simulink model "MRAC_Gradiet_LS_Algorithm_Ex8"  (R2023a)
settings: Solver=VariableStepAuto  StartTime=0.0  StopTime=20.0  RelTol=1e-13  AbsTol=1e-10
undefined symbols (not defined in the file): a, b, gamma1, gamma2, r0, r1
libraries: dspinverses x1, dspfactors x1
settings Model: Creator=geokr  LastModifiedBy=geokr

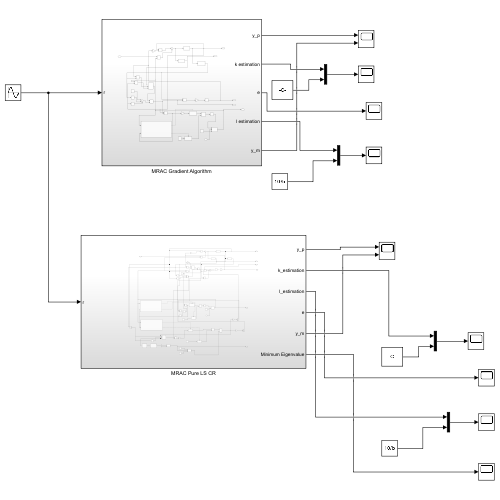
[thumbnail: Simulink's stored preview of the top-level diagram]
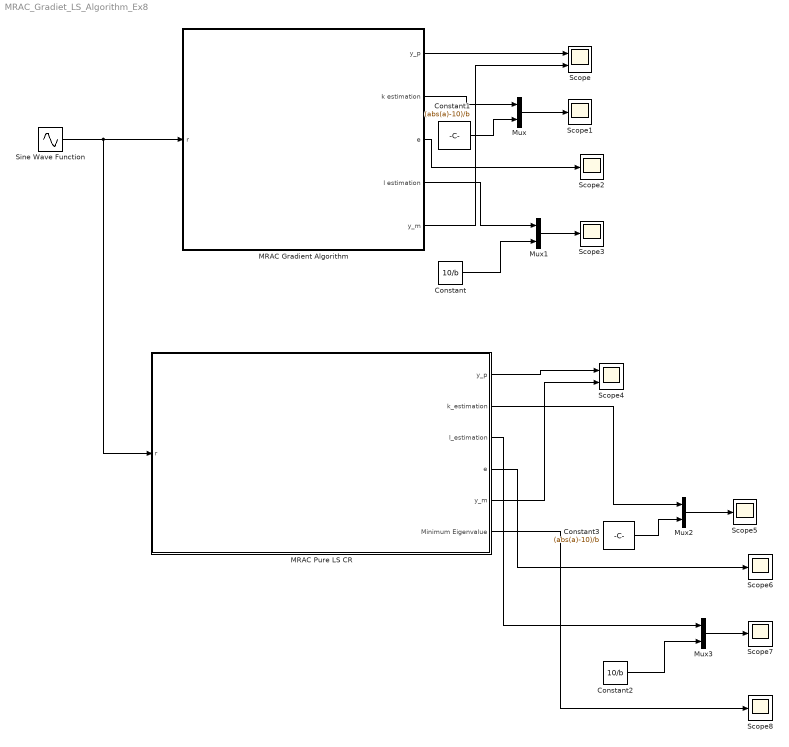
== system MRAC_Gradiet_LS_Algorithm_Ex8 ==
  Constant : Constant  Value=10/b
  Constant1 : Constant  Value=(abs(a)-10)/b
  Constant2 : Constant  Value=10/b
  Constant3 : Constant  Value=(abs(a)-10)/b
  MRAC Gradient Algorithm : Subsystem
  MRAC Pure LS CR : Subsystem
  Mux{,1..3} (4 alike) : Mux  Inputs=2
  Scope : Scope  NumInputPorts=2
  Scope{1..3,5..8} (7 alike) : Scope
  Scope4 : Scope  NumInputPorts=2
  Sine Wave Function : Sin  Frequency=2  SampleTime=0
  wires:
  MRAC Gradient Algorithm/1(y_p) -> Scope/1
  MRAC Gradient Algorithm/3(e) -> Scope2/1
  Mux/1 -> Scope1/1
  Mux1/1 -> Scope3/1
  MRAC Gradient Algorithm/2(k estimation) -> Mux/1
  MRAC Gradient Algorithm/4(l estimation) -> Mux1/1
  Constant/1 -> Mux1/2
  Constant1/1 -> Mux/2
  Sine Wave Function/1 -> MRAC Pure LS CR/1(r), MRAC Gradient Algorithm/1(r)
  MRAC Gradient Algorithm/5(y_m) -> Scope/2
  MRAC Pure LS CR/1(y_p) -> Scope4/1
  Constant3/1 -> Mux2/2
  Mux2/1 -> Scope5/1
  MRAC Pure LS CR/2(k_estimation) -> Mux2/1
  Mux3/1 -> Scope7/1
  Constant2/1 -> Mux3/2
  MRAC Pure LS CR/3(l_estimation) -> Mux3/1
  MRAC Pure LS CR/5(y_m) -> Scope4/2
  MRAC Pure LS CR/4(e) -> Scope6/1
  MRAC Pure LS CR/6(Minimum Eigenvalue) -> Scope8/1

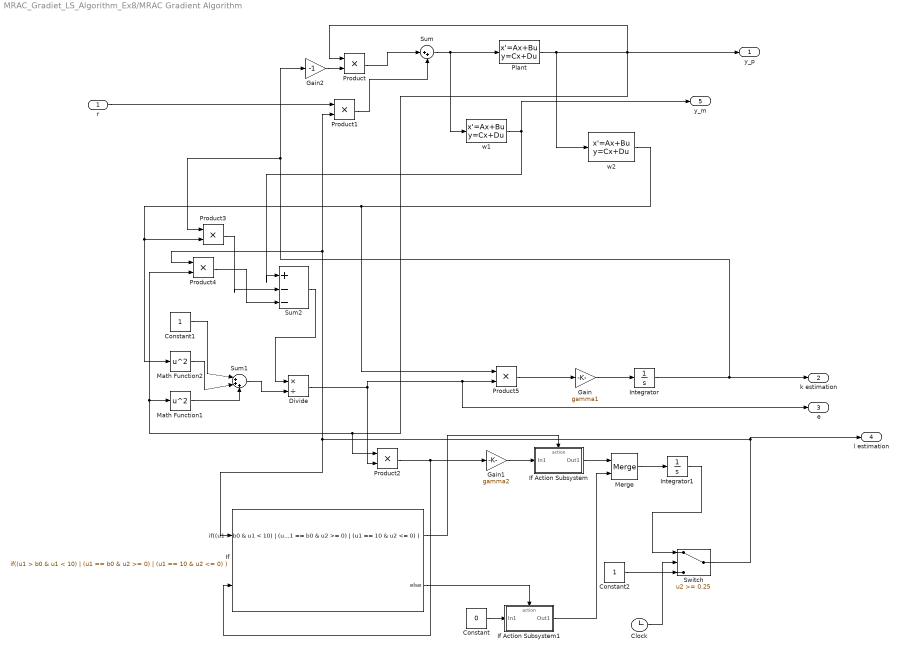
== system MRAC_Gradiet_LS_Algorithm_Ex8/MRAC Gradient Algorithm ==
  r : Inport
  Clock : Clock
  Constant : Constant  Value=0
  Constant1 : Constant
  Constant2 : Constant
  Divide : Product  Inputs=*/
  Gain : Gain  Gain=gamma1
  Gain1 : Gain  Gain=gamma2
  Gain2 : Gain  Gain=-1
  If : If  NumInputs=2  IfExpression=(u1 > b0 & u1 < 10) | (u1 == b0 & u2 >= 0) | (u1 == 10 & u2 <= 0)
  If Action Subsystem : Subsystem  TreatAsAtomicUnit=on
  If Action Subsystem1 : Subsystem  TreatAsAtomicUnit=on
  Integrator : Integrator
  Integrator1 : Integrator
  Math Function1 : Math  Operator=square
  Math Function2 : Math  Operator=square
  Merge : Merge
  Plant : StateSpace  A=a  B=b  D=0  InitialCondition=0
  Product{,1..5} (6 alike) : Product
  Sum : Sum  Inputs=|++
  Sum1 : Sum  Inputs=|+++
  Sum2 : Sum  Inputs=|+--
  Switch : Switch  Threshold=0.25  SaturateOnIntegerOverflow=off  InputSameDT=off
  w1 : StateSpace  A=-10  B=10  D=0  InitialCondition=0
  w2 : StateSpace  A=-10  B=10  D=0  InitialCondition=0
  y_p : Outport
  k estimation : Outport  Port=2
  e : Outport  Port=3
  l estimation : Outport  Port=4
  y_m : Outport  Port=5
  wires:
  If Action Subsystem/1(Out1) -> Merge/1
  Product2/1 -> If/2, Gain1/1
  Math Function2/1 -> Sum1/2
  Product/1 -> Sum/1
  w2/1 -> Math Function2/1, Product3/2, Product5/1
  Plant/1 -> w2/1, Product2/1, Product4/2, Math Function1/1, y_p/1, Product/1
  r/1 -> Product1/1
  Sum/1 -> w1/1, Plant/1
  Gain/1 -> Integrator/1
  Constant/1 -> If Action Subsystem1/1(In1)
  Math Function1/1 -> Sum1/3
  Product1/1 -> Sum/2
  w1/1 -> y_m/1, Sum2/1
  Gain1/1 -> If Action Subsystem/1(In1)
  If/2 -> If Action Subsystem1/Action
  Product3/1 -> Sum2/2
  If/1 -> If Action Subsystem/Action
  If Action Subsystem1/1(Out1) -> Merge/2
  Constant1/1 -> Sum1/1
  Product4/1 -> Sum2/3
  Sum1/1 -> Divide/2
  Product5/1 -> Gain/1
  Clock/1 -> Switch/2
  Merge/1 -> Integrator1/1
  Switch/1 -> If/1, Product4/1, Product1/2, l estimation/1
  Constant2/1 -> Switch/3
  Integrator1/1 -> Switch/1
  Integrator/1 -> k estimation/1, Gain2/1, Product3/1
  Sum2/1 -> Divide/1
  Divide/1 -> Product2/2, Product5/2, e/1
  Gain2/1 -> Product/2

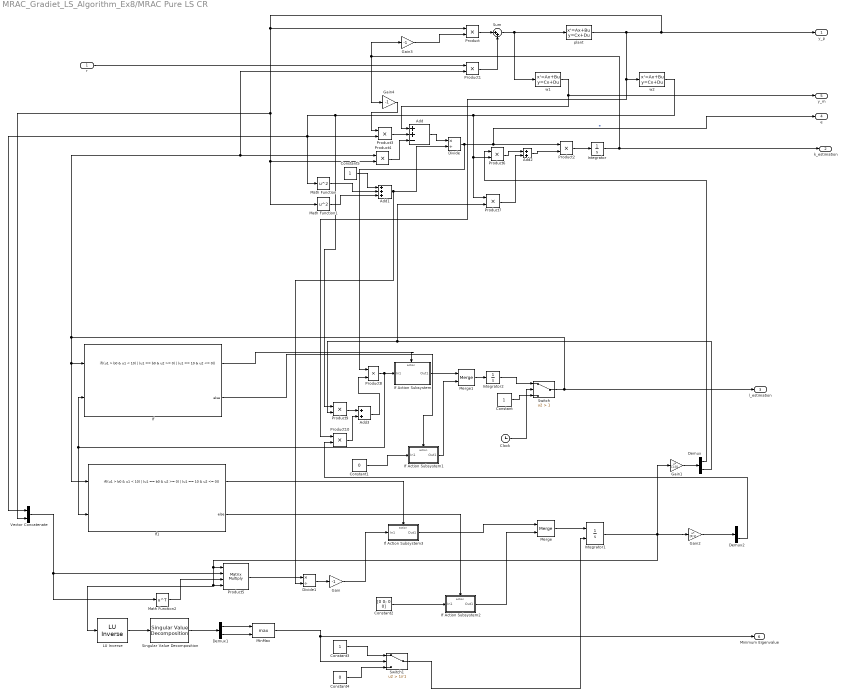
== system MRAC_Gradiet_LS_Algorithm_Ex8/MRAC Pure LS CR ==
  r : Inport
  " LU Inverse" : dspinverses/ LU Inverse
  Add : Sum  Inputs=++-
  Add1 : Sum  Inputs=+++
  Add2 : Sum
  Add3 : Sum
  Clock : Clock
  Constant : Constant
  Constant1 : Constant  Value=0
  Constant2 : Constant  Value=[0 0; 0 0]
  Constant3 : Constant
  Constant4 : Constant  Value=0
  Constant5 : Constant
  Demux : Demux  Outputs=2
  Demux1 : Demux  Outputs=2
  Demux2 : Demux  Outputs=2
  Divide : Product  Inputs=*/
  Divide1 : Product  Inputs=*/
  Gain : Gain  Gain=-1
  Gain1 : Gain  Gain=[1;0]  Multiplication=Matrix(u*K)
  Gain2 : Gain  Gain=[0;1]  Multiplication=Matrix(u*K)
  Gain3 : Gain  Gain=-1
  Gain4 : Gain  Gain=-1
  If : If  NumInputs=2  IfExpression=(u1 > b0 & u1 < 10) | (u1 == b0 & u2 >= 0) | (u1 == 10 & u2 <= 0)
  If Action Subsystem : Subsystem  TreatAsAtomicUnit=on
  If Action Subsystem1 : Subsystem  TreatAsAtomicUnit=on
  If Action Subsystem2 : Subsystem  TreatAsAtomicUnit=on
  If Action Subsystem3 : Subsystem  TreatAsAtomicUnit=on
  If1 : If  NumInputs=2  IfExpression=(u1 > b0 & u1 < 10) | (u1 == b0 & u2 >= 0) | (u1 == 10 & u2 <= 0)
  Integrator : Integrator
  Integrator1 : Integrator  ExternalReset=rising  InitialCondition=diag([r0 r0])
  Integrator2 : Integrator
  Math Function : Math  Operator=square
  Math Function1 : Math  Operator=square
  Math Function2 : Math  Operator=transpose
  Merge : Merge
  Merge1 : Merge
  MinMax : MinMax  Function=max  Inputs=2
  Product{,1..4,6..10} (10 alike) : Product
  Product5 : Product  Inputs=4  Multiplication=Matrix(*)
  Singular Value Decomposition : dspfactors/Singular Value Decomposition  wantv=on  wanterr=off  SimulateUsing=Interpreted execution
  Sum : Sum  Inputs=|++
  Switch : Switch  Criteria=u2 > Threshold  Threshold=1  SaturateOnIntegerOverflow=off  InputSameDT=off
  Switch1 : Switch  Criteria=u2 > Threshold  Threshold=1/r1  SaturateOnIntegerOverflow=off  InputSameDT=off
  Vector Concatenate : Concatenate
  plant : StateSpace  A=a  B=b  D=0  InitialCondition=0
  w1 : StateSpace  A=-10  B=10  D=0  InitialCondition=0
  w2 : StateSpace  A=-10  B=10  D=0  InitialCondition=0
  y_p : Outport
  k_estimation : Outport  Port=2
  l_estimation : Outport  Port=3
  e : Outport  Port=4
  y_m : Outport  Port=5
  Minimum Eigenvalue : Outport  Port=6
  wires:
  Product/1 -> Sum/1
  Product1/1 -> Sum/2
  Sum/1 -> w1/1, plant/1
  plant/1 -> Product10/1, w2/1, y_p/1, Product/1, Vector Concatenate/2, Math Function1/1, Product4/2
  r/1 -> Product1/1
  Integrator/1 -> k_estimation/1, Gain3/1, Gain4/1
  Product2/1 -> Integrator/1
  If1/2 -> If Action Subsystem2/Action
  If/2 -> If Action Subsystem1/Action
  If Action Subsystem2/1(Out1) -> Merge/2
  If Action Subsystem3/1(Out1) -> Merge/1
  If Action Subsystem1/1(Out1) -> Merge1/2
  If Action Subsystem/1(Out1) -> Merge1/1
  If/1 -> If Action Subsystem/Action
  If1/1 -> If Action Subsystem3/Action
  Merge1/1 -> Integrator2/1
  Integrator2/1 -> Switch/1
  Constant/1 -> Switch/3
  Switch/1 -> l_estimation/1, Product4/1, Product1/2, If1/1, If/1
  Constant1/1 -> If Action Subsystem1/1(In1)
  w1/1 -> y_m/1, Add/1
  Product3/1 -> Add/2
  Product4/1 -> Add/3
  Merge/1 -> Integrator1/1
  w2/1 -> Product7/1, Product6/2, Product9/1, Vector Concatenate/1, Product3/2, Math Function/1
  Math Function1/1 -> Add1/3
  Math Function/1 -> Add1/2
  Add/1 -> Divide/1
  Add1/1 -> Divide1/2, Divide/2
  Divide/1 -> Product8/1, Product2/1, e/1  "e"
  Constant4/1 -> Switch1/3
  Demux1/2 -> MinMax/2
  MinMax/1 -> Switch1/2, Minimum Eigenvalue/1
  Singular Value Decomposition/2 -> Demux1/1
  Demux1/1 -> MinMax/1
  Constant3/1 -> Switch1/1
  Switch1/1 -> Integrator1/2
  Vector Concatenate/1 -> Product5/2, Math Function2/1
  Math Function2/1 -> Product5/3
  Constant2/1 -> If Action Subsystem2/1(In1)
  Gain1/1 -> Demux/1
  Add2/1 -> Product2/2
  Product6/1 -> Add2/1
  Demux/1 -> Product6/1
  Demux/2 -> Product9/2, Product7/2
  Gain2/1 -> Demux2/1
  Product8/1 -> If/2, If1/2, If Action Subsystem/1(In1)
  Add3/1 -> Product8/2
  Product9/1 -> Add3/1
  Product10/1 -> Add3/2
  Demux2/2 -> Product10/2
  Constant5/1 -> Add1/1
  Clock/1 -> Switch/2
  " LU Inverse"/1 -> Singular Value Decomposition/1
  Gain3/1 -> Product/2
  Integrator1/1 -> " LU Inverse"/1, Product5/4, Product5/1, Gain2/1, Gain1/1
  Gain/1 -> If Action Subsystem3/1(In1)
  Divide1/1 -> Gain/1
  Product5/1 -> Divide1/1
  Product7/1 -> Add2/2
  Gain4/1 -> Product3/1

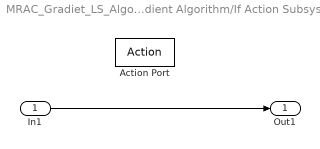
== system MRAC_Gradiet_LS_Algorithm_Ex8/MRAC Gradient Algorithm/If Action Subsystem ==
  In1 : Inport
  Action Port : ActionPort  ActionPortLabel=if((u1 > b0 & u1 < 10) | (u1 == b0 & u2 >= 0) | (u1 == 10 & u2 <= 0) )
  Out1 : Outport
  wires:
  In1/1 -> Out1/1

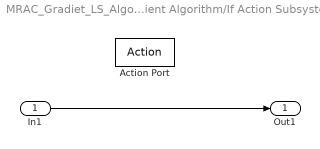
== system MRAC_Gradiet_LS_Algorithm_Ex8/MRAC Gradient Algorithm/If Action Subsystem1 ==
  In1 : Inport
  Action Port : ActionPort  ActionPortLabel=else
  Out1 : Outport
  wires:
  In1/1 -> Out1/1

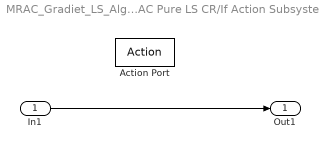
== system MRAC_Gradiet_LS_Algorithm_Ex8/MRAC Pure LS CR/If Action Subsystem ==
  In1 : Inport
  Action Port : ActionPort  ActionPortLabel=if((u1 > b0 & u1 < 10) | (u1 == b0 & u2 >= 0) | (u1 == 10 & u2 <= 0))
  Out1 : Outport
  wires:
  In1/1 -> Out1/1

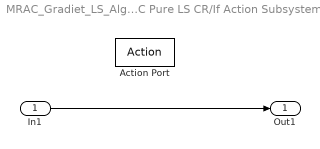
== system MRAC_Gradiet_LS_Algorithm_Ex8/MRAC Pure LS CR/If Action Subsystem1 ==
  In1 : Inport
  Action Port : ActionPort  ActionPortLabel=else
  Out1 : Outport
  wires:
  In1/1 -> Out1/1

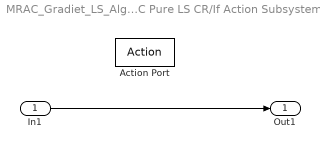
== system MRAC_Gradiet_LS_Algorithm_Ex8/MRAC Pure LS CR/If Action Subsystem2 ==
  In1 : Inport
  Action Port : ActionPort  ActionPortLabel=else
  Out1 : Outport
  wires:
  In1/1 -> Out1/1

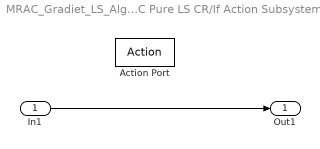
== system MRAC_Gradiet_LS_Algorithm_Ex8/MRAC Pure LS CR/If Action Subsystem3 ==
  In1 : Inport
  Action Port : ActionPort  ActionPortLabel=if((u1 > b0 & u1 < 10) | (u1 == b0 & u2 >= 0) | (u1 == 10 & u2 <= 0))
  Out1 : Outport
  wires:
  In1/1 -> Out1/1
